simulink model "untitled"  (R2020a)
settings: Solver=VariableStepAuto  StartTime=0.0  StopTime=10.0  RelTol=1e-3
settings Model: Creator=Kundan Patil  LastModifiedBy=Kundan Patil

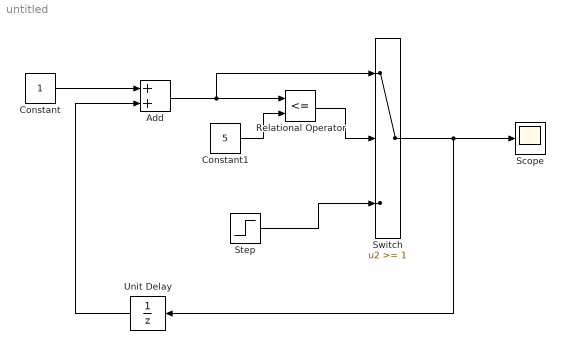
== system untitled ==
  Add : Sum
  Constant : Constant
  Constant1 : Constant  Value=5
  Relational Operator : RelationalOperator  Operator=<=  OutDataTypeStr=boolean  RndMeth=Simplest
  Scope : Scope
  Step : Step  Before=-5  After=0  SampleTime=0
  Switch : Switch  Threshold=1
  Unit Delay : UnitDelay  InitialCondition=-1  SampleTime=-1  HasFrameUpgradeWarning=on
  wires:
  Constant/1 -> Add/1
  Constant1/1 -> Relational Operator/2
  Add/1 -> Switch/1, Relational Operator/1
  Relational Operator/1 -> Switch/2
  Unit Delay/1 -> Add/2
  Step/1 -> Switch/3
  Switch/1 -> Unit Delay/1, Scope/1
